simulink model "poleplace_luenburg_roo"  (Simulink 7.5)
settings: Solver=ode4  StartTime=0.0  StopTime=3.1  FixedStep=0.001  RelTol=1e-3
PreLoadFcn:
  | poleplace_luenburg_roo_param
values from neighbouring files (symbols this model uses):
  A_ = inv_T * A * T,    [poleplace_luenburg_roo_param.m]
  AA = A11 - G*A21,    [poleplace_luenburg_roo_param.m]    (also in poleplace_sfb_luenburg_roo_param.m = Abb - G*Aab,)
  B_ = inv_T * B,    [poleplace_luenburg_roo_param.m]
  BB = B_1 - G*B_2,    [poleplace_luenburg_roo_param.m]    (also in poleplace_sfb_luenburg_roo_param.m = Bb - G*Ba,)
  C_ = C * T,    [poleplace_luenburg_roo_param.m]
  G = phi_A*inv(N)*[0; 1]    [poleplace_luenburg_foo_param.m]    (also in poleplace_luenburg_roo_param.m = acker(A11', A21',  pole_esti_desired )',; poleplace_sfb_luenburg_foo_param.m = acker(A', C', p)'; poleplace_sfb_luenburg_roo_param.m = acker(Abb', Aab',  pole_esti_desired )',)
  GG = (A11 - G*A21)*G + (A12-G*A22),    [poleplace_luenburg_roo_param.m]    (also in poleplace_sfb_luenburg_roo_param.m = (Abb - G*Aab)*G + (Aba - G*Aaa),)
settings Model: Creator=Huiliang  LastModifiedBy=Dell
settings OptimizationCC: InitFltsAndDblsToZero=on
settings DebuggingCC: SaveWithParameterizedLinksMsg=none  StrictBusMsg=Warning
settings GRTTargetCC: TargetFcnLib=ansi_tfl_tmw.mat

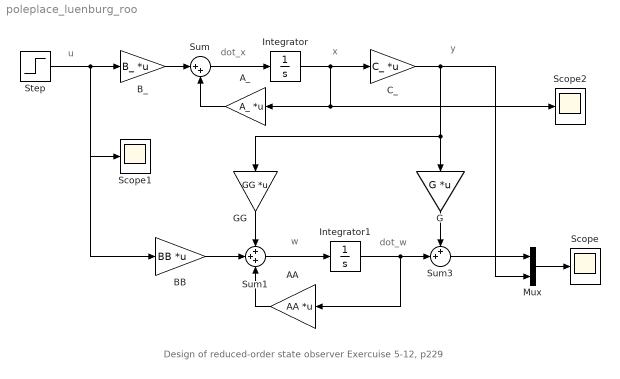
== system poleplace_luenburg_roo ==
  note: x
  note: dot_x
  note: y
  note: u
  note: w
  note: dot_w
  note: Design of reduced-order state observer
      | Exercuise 5-12, p229
  AA : Gain  Gain=AA  Multiplication=Matrix(K*u)  ParameterDataType=sfix(16)  ParameterScaling=2^0  OutDataType=sfix(16)  OutScaling=2^0
  A_ : Gain  Gain=A_  Multiplication=Matrix(K*u)  ParameterDataType=sfix(16)  ParameterScaling=2^0  OutDataType=sfix(16)  OutScaling=2^0
  BB : Gain  Gain=BB  Multiplication=Matrix(K*u)  ParameterDataType=sfix(16)  ParameterScaling=2^0  OutDataType=sfix(16)  OutScaling=2^0
  B_ : Gain  Gain=B_  Multiplication=Matrix(K*u)  ParameterDataType=sfix(16)  ParameterScaling=2^0  OutDataType=sfix(16)  OutScaling=2^0
  C_ : Gain  Gain=C_  Multiplication=Matrix(K*u)  ParameterDataType=sfix(16)  ParameterScaling=2^0  OutDataType=sfix(16)  OutScaling=2^0
  G : Gain  Gain=G  Multiplication=Matrix(K*u)  ParameterDataType=sfix(16)  ParameterScaling=2^0  OutDataType=sfix(16)  OutScaling=2^0
  GG : Gain  Gain=GG  Multiplication=Matrix(K*u)  ParameterDataType=sfix(16)  ParameterScaling=2^0  OutDataType=sfix(16)  OutScaling=2^0
  Integrator : Integrator  InitialCondition="[-0.01;   0.01;  0 ]"
  Integrator1 : Integrator  InitialCondition="[0;    0]"
  Mux : Mux  Inputs=2
  Scope : Scope
      settings: TimeRange=3.5  YMin=-0.04  YMax=0.1
  Scope1 : Scope
      settings: TimeRange=6  YMin=-1  YMax=1
  Scope2 : Scope
      settings: TimeRange=3.5  YMin=-0.04  YMax=0.1  SaveName=ScopeData2
  Step : Step  Time=3  SampleTime=0
  Sum : Sum  Inputs=|++  OutDataType=sfix(16)  OutScaling=2^0
  Sum1 : Sum  Inputs=+++  OutDataType=sfix(16)  OutScaling=2^0
  Sum3 : Sum  Inputs=++|  OutDataType=sfix(16)  OutScaling=2^0
  wires:
  Integrator/1 -> C_/1, A_/1, Scope2/1
  Sum/1 -> Integrator/1
  B_/1 -> Sum/1
  C_/1 -> GG/1, G/1, Mux/2
  BB/1 -> Sum1/2
  Sum1/1 -> Integrator1/1
  Integrator1/1 -> AA/1, Sum3/2
  Mux/1 -> Scope/1
  G/1 -> Sum3/1
  GG/1 -> Sum1/1
  AA/1 -> Sum1/3
  A_/1 -> Sum/2
  Step/1 -> B_/1, BB/1, Scope1/1
  Sum3/1 -> Mux/1
